simulink model "ModulationUnit"  (R2023a)
settings: Solver=FixedStepAuto  StartTime=0.0  StopTime=20  FixedStep=0.0001  MaxStep=1e-5  RelTol=1e-3  AbsTol=1e-3
settings Model: PacingRate=1000  Creator=ykamatan  LastModifiedBy=ykamatan
settings SolverCC: AutoScaleAbsTol=off  SolverJacobianMethodControl=SparsePerturbation  DaesscMode=Fast
settings DataIOCC: SaveOutput=off  SaveTime=off
settings OptimizationCC: ReuseModelBlockBuffer=off
settings DebuggingCC: UnconnectedInputMsg=warning  UnconnectedOutputMsg=warning  UnconnectedLineMsg=warning  SymbolicDimsDataTypeCodeGenerationDiagnostic=none
settings ModelReferenceCC: EnableRefExpFcnMdlSchedulingChecks=on
settings SFSimCC: CustomCodeUndefinedFunction=UseInterfaceOnly
settings RTWCC: DLArmComputeVersion=19.05
settings SimscapeCC: SimscapeLogDataHistory=10000

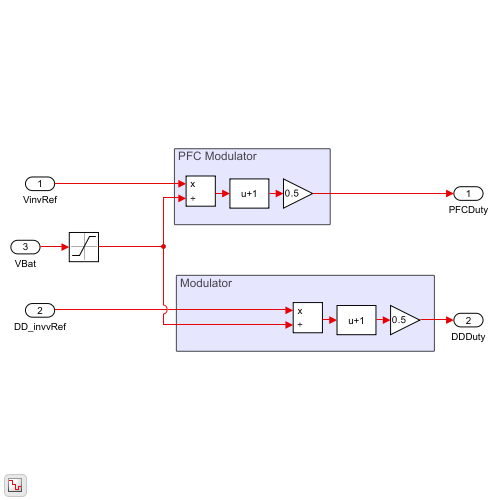
[thumbnail: Simulink's stored preview of the top-level diagram]
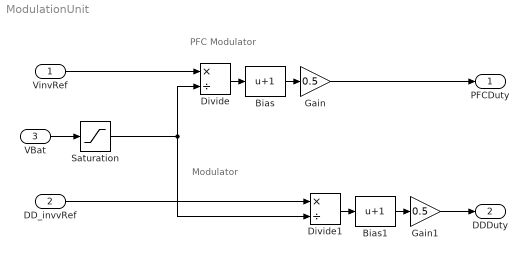
== system ModulationUnit ==
  note: Modulator
  note: PFC Modulator
  VinvRef : Inport  OutDataTypeStr=double  PortDimensions=1  SampleTime=[0.0001,0]
  DD_invvRef : Inport  Port=2  OutDataTypeStr=double  PortDimensions=1  SampleTime=[0.0001,0]
  VBat : Inport  Port=3
  Bias : Bias  Bias=1  SaturateOnIntegerOverflow=off
  Bias1 : Bias  Bias=1  SaturateOnIntegerOverflow=off
  Divide : Product  Inputs=*/
  Divide1 : Product  Inputs=*/
  Gain : Gain  Gain=0.5
  Gain1 : Gain  Gain=0.5
  Saturation : Saturate  UpperLimit=inf  LowerLimit=10
  PFCDuty : Outport  OutDataTypeStr=double  PortDimensions=1  SampleTime=[0.0001,0]
  DDDuty : Outport  Port=2  OutDataTypeStr=double  PortDimensions=1  SampleTime=[0.0001,0]
  wires:
  Gain/1 -> PFCDuty/1
  VBat/1 -> Saturation/1
  Divide/1 -> Bias/1
  Bias/1 -> Gain/1
  VinvRef/1 -> Divide/1
  Saturation/1 -> Divide1/2, Divide/2
  Gain1/1 -> DDDuty/1
  Divide1/1 -> Bias1/1
  Bias1/1 -> Gain1/1
  DD_invvRef/1 -> Divide1/1
